simulink model "RL_sus_quarter_sim"  (R2025a)
settings: Solver=FixedStepAuto  StartTime=0.0  StopTime=20  FixedStep=0.001  RelTol=1e-3
model workspace (MAT data in the model file):
  G0 : Simulink.Parameter (value not decoded)
  Q_F : Simulink.Parameter (value not decoded)
  Q_dot_s : Simulink.Parameter (value not decoded)
  Q_dot_s_h : Simulink.Parameter (value not decoded)
  Q_dot_u : Simulink.Parameter (value not decoded)
  Q_flec : Simulink.Parameter (value not decoded)
  Q_flec_t : Simulink.Parameter (value not decoded)
  b_deflec : Simulink.Parameter (value not decoded)
  bump_height : Simulink.Parameter (value not decoded)
  bump_lenth : Simulink.Parameter (value not decoded)
  bump_start : Simulink.Parameter (value not decoded)
  f0 : Simulink.Parameter (value not decoded)
  kt : Simulink.Parameter (value not decoded)
  ms : Simulink.Parameter (value not decoded)
  n0 : Simulink.Parameter (value not decoded)
  n1 : Simulink.Parameter (value not decoded)
  omega_1 : Simulink.Parameter (value not decoded)
  omega_2 : Simulink.Parameter (value not decoded)
  omega_3 : Simulink.Parameter (value not decoded)
  omega_4 : Simulink.Parameter (value not decoded)
  ramp_height : Simulink.Parameter (value not decoded)
  ramp_lenth : Simulink.Parameter (value not decoded)
  ramp_start : Simulink.Parameter (value not decoded)
  sine_amp : Simulink.Parameter (value not decoded)
  sine_freq : Simulink.Parameter (value not decoded)
  u : Simulink.Parameter (value not decoded)
symbols that are objects in the model workspace (value not decoded): b_deflec, bump_height, bump_lenth, bump_start, f0, G0, kt, ms, n0, n1, omega_1, omega_2, omega_3, omega_4, Q_dot_s, Q_dot_s_h, Q_F, Q_flec, Q_flec_t, ramp_height, ramp_lenth, ramp_start, sine_amp, sine_freq
undefined symbols (not defined in the file): Ground, Hook, SH_ADD_new_as_as_xdef
libraries: fl_lib x250, nesl_utility x48, sharedTrackingLibrary x34, dspstat3 x18, simulink x3, deeplib x2, slpidlib x1
(part 7 of 12)

== system RL_sus_quarter_sim/Quarter_sys/Control/Y_1/freq semi/Subsystem2 ==
  v_def : Inport
  x_def : Inport  Port=2
  Add1 : Sum
  Gain : Gain  Gain=-1
  Lmbada_C : Constant  Value=1000
  Product1 : Product
  ks : Gain  Gain=-20000
  Out1 : Outport
  wires:
  ks/1 -> Add1/2
  x_def/1 -> ks/1
  Product1/1 -> Gain/1
  Lmbada_C/1 -> Product1/2
  Gain/1 -> Add1/1
  v_def/1 -> Product1/1
  Add1/1 -> Out1/1

== system RL_sus_quarter_sim/Quarter_sys/Control/Y_1/freq semi/Subsystem3 ==
  v_def : Inport
  x_def : Inport  Port=2
  Add1 : Sum
  Gain : Gain  Gain=-1
  Lmbada_C : Constant  Value=2000
  Product1 : Product
  ks : Gain  Gain=-20000
  Out1 : Outport
  wires:
  Add1/1 -> Out1/1
  v_def/1 -> Product1/1
  Gain/1 -> Add1/1
  Lmbada_C/1 -> Product1/2
  Product1/1 -> Gain/1
  x_def/1 -> ks/1
  ks/1 -> Add1/2

== system RL_sus_quarter_sim/Quarter_sys/Control/Y_1/imp_force_RL_model/Subsystem ==
  v_s : Inport
  Abs : Abs  SaturateOnIntegerOverflow=off
  Chart : Stateflow chart  TreatAsAtomicUnit=on  SystemSampleTime=0.001
  Chart1 : Stateflow chart  TreatAsAtomicUnit=on  SystemSampleTime=0.001
  Constant : Constant  Value=10000
  Constant1 : Constant  Value=10
  Constant2 : Constant  Value=1000
  Constant3 : Constant  Value=-500
  Constant4 : Constant  Value=-10000
  Constant5 : Constant  Value=30
  Constant6 : Constant  Value=3
  Constant8 : Constant  Value=0
  Demux : Demux  Outputs=2
  FS1 : Constant  Value=0.65
  FS2 : Constant  Value=4.5
  L1 : Subsystem
  L2 : Subsystem
  L3 : Subsystem
  MATLAB Function2 : Subsystem  Variant=on  VariantControlMode=label  VariantControl=MATLAB Function1  LabelModeActiveChoice=adaptive IFEKF simple
  Manual Switch : ManualSwitch
  Multiport Switch : MultiPortSwitch  Inputs=2  SaturateOnIntegerOverflow=off  InputSameDT=off
  Multiport Switch1 : MultiPortSwitch  Inputs=7  SaturateOnIntegerOverflow=off  InputSameDT=off
  Mux : Mux
  Mux1 : Mux  Inputs=2
  Mux2 : Mux  Inputs=2
  Scope : Scope
      settings: ActiveDisplayYMinimum=7.5  ActiveDisplayYMaximum=32.5
  Scope1 : Scope
      settings: ActiveDisplayYMinimum=-10696.7424  ActiveDisplayYMaximum=10249.86115  DataLoggingVariableName=ScopeData2
  Scope2 : Scope
      settings: ActiveDisplayYMinimum=0.875  ActiveDisplayYMaximum=2.125  DataLoggingVariableName=ScopeData3
  Zero-Order Hold : ZeroOrderHold  SampleTime=0.001
  passive : Subsystem
  Out1 : Outport
  wires:
  Constant8/1 -> MATLAB Function2/2(epsilon)
  Zero-Order Hold/1 -> MATLAB Function2/1(y)
  MATLAB Function2/6(omega) -> Abs/1
  v_s/1 -> Zero-Order Hold/1
  Abs/1 -> Chart/1(freq), Chart1/1(freq)
  FS1/1 -> Chart/2(FS1)
  FS2/1 -> Chart/3(FS2)
  Demux/1 -> Mux/1, Scope1/1  "k_a1"
  Constant3/1 -> Mux/2  "c_a1"
  Constant2/1 -> Mux/3  "c_a2"
  Demux/2 -> Scope/1, Mux/4  "b"
  Mux/1 -> ?
  Chart/1(level) -> Multiport Switch/1
  Multiport Switch/1 -> Demux/1
  Constant/1 -> Mux1/1  "ka1"
  Constant1/1 -> Mux1/2  "b"
  Mux1/1 -> Multiport Switch/2  "L1"
  Constant4/1 -> Mux2/1  "ka1"
  Constant5/1 -> Mux2/2  "b"
  Mux2/1 -> Multiport Switch/3  "L2"
  Chart1/1(level) -> Scope2/1, Manual Switch/1
  Multiport Switch1/1 -> Out1/1
  L1/1(Out1) -> Multiport Switch1/5, Multiport Switch1/8
  Manual Switch/1 -> Multiport Switch1/1
  Constant6/1 -> Manual Switch/2
  L3/1(Out1) -> Multiport Switch1/4, Multiport Switch1/7
  L2/1(Out1) -> Multiport Switch1/2, Multiport Switch1/3
  passive/1(Out1) -> Multiport Switch1/6

== system RL_sus_quarter_sim/Quarter_sys/Control/Y_1/imp_force_RL_model/bkkcc ==
  v_def : Inport
  x_def : Inport  Port=2
  a_def : Inport  Port=3
  param_ctr : Inport  Port=4
  Add : Sum  Inputs=+++
  Add1 : Sum
  Demux : Demux
  Divide : Product  Inputs=*/
  Gain{,1..3} (4 alike) : Gain  Gain=-1
  Integrator : Integrator
  Product{,1..3} (4 alike) : Product
  F_bkkcc : Outport
  wires:
  x_def/1 -> Product/2
  Demux/1 -> Gain/1  "k_a1"
  Product/1 -> Add/1
  Demux/2 -> Gain1/1  "c_a1"
  Product1/1 -> Add/2
  Add/1 -> F_bkkcc/1
  Demux/3 -> Product3/1, Gain2/1  "c_a2"
  Demux/4 -> Gain3/1  "b"
  Product2/1 -> Add/3
  Gain/1 -> Product/1
  Gain1/1 -> Product1/1
  Gain2/1 -> Product2/1
  Gain3/1 -> Divide/2
  param_ctr/1 -> Demux/1
  Add1/1 -> Integrator/1  "a1"
  Divide/1 -> Add1/1
  a_def/1 -> Add1/2
  v_def/1 -> Product1/2
  Integrator/1 -> Product2/2, Product3/2  "v1"
  Product3/1 -> Divide/1

== system RL_sus_quarter_sim/Quarter_sys/Passive/Y_1/P_0/Subsystem ==
  p0_k2 : Subsystem  VariantControl=p0_k2
  p0_k3 : Subsystem  VariantControl=p0_k3
  p0_k4 : Subsystem  VariantControl=p0_k4
  p0_k6 : Subsystem  VariantControl=p0_k6
  passive : Subsystem  VariantControl=passive
  Conn1 : PMIOPort  Side=Right
  Conn2 : PMIOPort  Port=2  Side=Left

== system RL_sus_quarter_sim/Quarter_sys/Passive/Y_1/P_1/Subsystem ==
  p1_k1 : Subsystem  VariantControl=p1_k1
  p1_k2 : Subsystem  VariantControl=p1_k2
  p1_k3 : Subsystem  VariantControl=p1_k3
  p1_k5 : Subsystem  VariantControl=p1_k5
  passive : Subsystem  VariantControl=passive
  Conn1 : PMIOPort  Side=Right
  Conn2 : PMIOPort  Port=2  Side=Left

== system RL_sus_quarter_sim/Quarter_sys/Passive/Y_1/P_test/Subsystem ==
  p1_k1 : Subsystem  VariantControl=p1_k1
  p1_k2 : Subsystem  VariantControl=p1_k2
  p1_k3 : Subsystem  VariantControl=p1_k3
  p1_k5 : Subsystem  VariantControl=p1_k5
  passive : Subsystem  VariantControl=passive
  Conn1 : PMIOPort  Side=Right
  Conn2 : PMIOPort  Port=2  Side=Left

== system RL_sus_quarter_sim/Quarter_sys/Passive/Y_1/Sky-Hook/Subsystem ==
  p1_k1 : Subsystem  VariantControl=p1_k1
  p1_k2 : Subsystem  VariantControl=p1_k2
  p1_k3 : Subsystem  VariantControl=p1_k3
  p1_k5 : Subsystem  VariantControl=p1_k5
  passive : Subsystem  VariantControl=passive
  Conn1 : PMIOPort  Side=Right
  Conn2 : PMIOPort  Port=2  Side=Left

== system RL_sus_quarter_sim/Quarter_sys/Control/Y_1/ADP_NN/reference/constant ==
  Add : Sum
  Constant : Constant  Value=0
  Constant1 : Constant  Value=0
  Constant2 : Constant  Value=sine_amp
  Manual Switch : ManualSwitch  CurrentSetting=0
  Repeating Sequence Stair : simulink/Sources/Repeating Sequence Stair  OutValues=[0 0.02].'  tsamp=3  OutMin=[]  OutMax=[]  OutDataTypeStr=double  OutputDataTypeScalingMode=double  OutDataType=fixdt(0,8)  ConRadixGroup=Best Precision: Vector-wise  OutScaling=2^-12
  xs_ref : Outport
  vs_ref : Outport  Port=2
  wires:
  Constant1/1 -> vs_ref/1
  Constant/1 -> Manual Switch/1
  Manual Switch/1 -> xs_ref/1
  Constant2/1 -> Add/1
  Repeating Sequence Stair/1 -> Add/2
  Add/1 -> Manual Switch/2

== system RL_sus_quarter_sim/Quarter_sys/Control/Y_1/ADP_NN/reference/skyhook_virtual ==
  xs : Inport
  vs : Inport  Port=2
  Add : Sum
  Add1 : Sum
  Add2 : Sum
  Divide : Product  Inputs=*/
  Product : Product
  Product1 : Product
  dt_v : Gain  Gain=0.1
  ms_v : Constant  Value=400
  skyhook_c : Constant  Value=-1000
  skyhook_k : Constant  Value=-10000
  xs_ref : Outport
  vs_ref : Outport  Port=2
  wires:
  xs/1 -> Add1/2, Product/1
  skyhook_k/1 -> Product/2
  vs/1 -> Add2/2, Product1/1
  skyhook_c/1 -> Product1/2
  Product/1 -> Add/1
  Product1/1 -> Add/2
  Add/1 -> Divide/1  "F_skyhook_v"
  ms_v/1 -> Divide/2
  Divide/1 -> dt_v/1  "skyhook_as_v"
  dt_v/1 -> Add2/1, Add1/1
  Add1/1 -> xs_ref/1
  Add2/1 -> vs_ref/1

== system RL_sus_quarter_sim/Quarter_sys/Control/Y_1/Freq_imp/Low_with_Alpha/Subsystem ==
  p1_k1 : Subsystem  VariantControl=p1_k1
  p1_k2 : Subsystem  VariantControl=p1_k2
  p1_k3 : Subsystem  VariantControl=p1_k3
  p1_k5 : Subsystem  VariantControl=p1_k5
  passive : Subsystem  VariantControl=passive
  Conn1 : PMIOPort  Side=Right
  Conn2 : PMIOPort  Port=2  Side=Left

== system RL_sus_quarter_sim/Quarter_sys/Control/Y_1/Freq_imp/high_with_Alpha/Subsystem ==
  p1_k1 : Subsystem  VariantControl=p1_k1
  p1_k2 : Subsystem  VariantControl=p1_k2
  p1_k3 : Subsystem  VariantControl=p1_k3
  p1_k5 : Subsystem  VariantControl=p1_k5
  passive : Subsystem  VariantControl=passive
  Conn1 : PMIOPort  Side=Right
  Conn2 : PMIOPort  Port=2  Side=Left

== system RL_sus_quarter_sim/Quarter_sys/Control/Y_1/Freq_imp1/Low_with_Alpha/Subsystem ==
  p1_k1 : Subsystem  VariantControl=p1_k1
  p1_k2 : Subsystem  VariantControl=p1_k2
  p1_k3 : Subsystem  VariantControl=p1_k3
  p1_k5 : Subsystem  VariantControl=p1_k5
  passive : Subsystem  VariantControl=passive
  Conn1 : PMIOPort  Side=Right
  Conn2 : PMIOPort  Port=2  Side=Left

== system RL_sus_quarter_sim/Quarter_sys/Control/Y_1/Freq_imp1/Subsystem/2nd_FS ==
  vs : Inport
  au : Inport  Port=2
  alpha : Inport  Port=3
  2nd_FS : Sum  Inputs=+-
  Constant4 : Constant  Value=20000
  Constant5 : Constant  Value=400
  Constant6 : Constant  Value=1000
  Gain : Gain  Gain=2*pi
  MATLAB Function1 : MATLAB Function  TreatAsAtomicUnit=on
  Product : Product
  Square : Math  Operator=square
  Square1 : Math  Operator=square
  FS2 : Outport
  wires:
  Gain/1 -> Square/1, MATLAB Function1/2(alpha)
  Square/1 -> Product/1
  Constant5/1 -> MATLAB Function1/4(ms)
  2nd_FS/1 -> FS2/1
  MATLAB Function1/1(y) -> 2nd_FS/1
  Constant6/1 -> MATLAB Function1/5(cs)
  Constant4/1 -> MATLAB Function1/3(ks)
  Product/1 -> 2nd_FS/2
  au/1 -> MATLAB Function1/1(au)
  vs/1 -> Square1/1
  Square1/1 -> Product/2
  alpha/1 -> Gain/1

== system RL_sus_quarter_sim/Quarter_sys/Control/Y_1/Freq_imp1/Subsystem/FS1 ==
  vs : Inport
  au : Inport  Port=2
  alpha : Inport  Port=3
  2nd_FS : Sum  Inputs=+-
  Constant4 : Constant  Value=20000
  Constant5 : Constant  Value=400
  Constant6 : Constant  Value=1000
  Gain : Gain  Gain=2*pi
  MATLAB Function1 : MATLAB Function  TreatAsAtomicUnit=on
  Product : Product
  Scope : Scope  NumInputPorts=2
      settings: ActiveDisplayYMinimum=-2.36691  ActiveDisplayYMaximum=3.61329  DataLoggingVariableName=ScopeData8
  Square : Math  Operator=square
  Square1 : Math  Operator=square
  FS2 : Outport
  wires:
  Square1/1 -> Product/2
  vs/1 -> Square1/1
  au/1 -> MATLAB Function1/1(au)
  Product/1 -> Scope/2, 2nd_FS/2
  Constant4/1 -> MATLAB Function1/3(ks)
  Constant6/1 -> MATLAB Function1/5(cs)
  MATLAB Function1/1(y) -> Scope/1, 2nd_FS/1
  2nd_FS/1 -> FS2/1
  Constant5/1 -> MATLAB Function1/4(ms)
  Square/1 -> Product/1
  Gain/1 -> MATLAB Function1/2(alpha), Square/1
  alpha/1 -> Gain/1

== system RL_sus_quarter_sim/Quarter_sys/Control/Y_1/Freq_imp1/high_with_Alpha/Subsystem ==
  p1_k1 : Subsystem  VariantControl=p1_k1
  p1_k2 : Subsystem  VariantControl=p1_k2
  p1_k3 : Subsystem  VariantControl=p1_k3
  p1_k5 : Subsystem  VariantControl=p1_k5
  passive : Subsystem  VariantControl=passive
  Conn1 : PMIOPort  Side=Right
  Conn2 : PMIOPort  Port=2  Side=Left

== system RL_sus_quarter_sim/Quarter_sys/Control/Y_1/IFEKF FDC/Subsystem/MATLAB Function2 ==
  y : Inport
  epsilon : Inport  Port=2
  EKF epsilon : Subsystem  VariantControl=Extended Kalman Filter habib epsilon
  EKF simple Amp : Subsystem  VariantControl=EKFhabib epsilon Amp
  IFEKF simple : Subsystem  VariantControl=IFEKF simple
  adaptive IFEKF sdimple_3 : Subsystem  VariantControl=adaptive IFEKF sdimple_3
  adaptive IFEKF simple : Subsystem  VariantControl=adaptive IFEKF simple
  x1hat : Outport
  P : Outport  Port=2
  debug : Outport  Port=3
  xhat_pred : Outport  Port=4
  y_residual : Outport  Port=5
  omega : Outport  Port=6

== system RL_sus_quarter_sim/Quarter_sys/Control/Y_1/IFEKF SHADD/Subsystem/MATLAB Function2 ==
  y : Inport
  epsilon : Inport  Port=2
  EKF epsilon : Subsystem  VariantControl=Extended Kalman Filter habib epsilon
  EKF simple Amp : Subsystem  VariantControl=EKFhabib epsilon Amp
  IFEKF simple : Subsystem  VariantControl=IFEKF simple
  adaptive IFEKF simple : Subsystem  VariantControl=adaptive IFEKF simple
  x1hat : Outport
  P : Outport  Port=2
  debug : Outport  Port=3
  xhat_pred : Outport  Port=4
  y_residual : Outport  Port=5
  omega : Outport  Port=6

== system RL_sus_quarter_sim/Quarter_sys/Control/Y_1/IFEKF Select c/Subsystem/MATLAB Function2 ==
  y : Inport
  epsilon : Inport  Port=2
  EKF epsilon : Subsystem  VariantControl=Extended Kalman Filter habib epsilon
  EKF simple Amp : Subsystem  VariantControl=EKFhabib epsilon Amp
  IFEKF simple : Subsystem  VariantControl=IFEKF simple
  adaptive IFEKF simple : Subsystem  VariantControl=adaptive IFEKF simple
  x1hat : Outport
  P : Outport  Port=2
  debug : Outport  Port=3
  xhat_pred : Outport  Port=4
  y_residual : Outport  Port=5
  omega : Outport  Port=6

== system RL_sus_quarter_sim/Quarter_sys/Control/Y_1/IFEKF Select c/Subsystem2/constant ==
  sig select : Inport
  v_def : Inport  Port=2
  Multiport Switch : MultiPortSwitch  SaturateOnIntegerOverflow=off  InputSameDT=off
  large C : Subsystem
  "mid C " : Subsystem
  small C : Subsystem
  F_damper : Outport
  wires:
  Multiport Switch/1 -> F_damper/1  "F_damper"
  small C/1(Out1) -> Multiport Switch/3
  large C/1(F_sus1) -> Multiport Switch/2
  "mid C "/1(Out1) -> Multiport Switch/4
  sig select/1 -> Multiport Switch/1
  v_def/1 -> large C/1(v_def), "mid C "/1(v_def), small C/1(v_def)

== system RL_sus_quarter_sim/Quarter_sys/Control/Y_1/IFEKF Select c/Subsystem2/semi ctr ==
  sig select : Inport
  v_def : Inport  Port=2
  v_s : Inport  Port=3
  a_s : Inport  Port=4
  ADD : Subsystem
  Multiport Switch : MultiPortSwitch  SaturateOnIntegerOverflow=off  InputSameDT=off
  SH : Subsystem
  Subsystem1 : Subsystem
  F_damper : Outport
  wires:
  v_s/1 -> SH/2(v_s)
  v_def/1 -> SH/1(v_def), Subsystem1/1(v_def), ADD/1(v_def)
  sig select/1 -> Multiport Switch/1
  Subsystem1/1(Out1) -> Multiport Switch/4
  ADD/1(F_sus1) -> Multiport Switch/3
  a_s/1 -> ADD/2(a_s)
  SH/1(Out1) -> Multiport Switch/2
  Multiport Switch/1 -> F_damper/1  "F_damper"

== system RL_sus_quarter_sim/Quarter_sys/Control/Y_1/IFEKF freq b/Subsystem/MATLAB Function2 ==
  y : Inport
  epsilon : Inport  Port=2
  EKF epsilon : Subsystem  VariantControl=Extended Kalman Filter habib epsilon
  EKF simple Amp : Subsystem  VariantControl=EKFhabib epsilon Amp
  IFEKF simple : Subsystem  VariantControl=IFEKF simple
  adaptive IFEKF simple : Subsystem  VariantControl=adaptive IFEKF simple
  x1hat : Outport
  P : Outport  Port=2
  debug : Outport  Port=3
  xhat_pred : Outport  Port=4
  y_residual : Outport  Port=5
  omega : Outport  Port=6

== system RL_sus_quarter_sim/Quarter_sys/Control/Y_1/IFEKF freq bc/Subsystem/MATLAB Function2 ==
  y : Inport
  epsilon : Inport  Port=2
  EKF epsilon : Subsystem  VariantControl=Extended Kalman Filter habib epsilon
  EKF simple Amp : Subsystem  VariantControl=EKFhabib epsilon Amp
  IFEKF simple : Subsystem  VariantControl=IFEKF simple
  adaptive IFEKF simple : Subsystem  VariantControl=adaptive IFEKF simple
  x1hat : Outport
  P : Outport  Port=2
  debug : Outport  Port=3
  xhat_pred : Outport  Port=4
  y_residual : Outport  Port=5
  omega : Outport  Port=6

== system RL_sus_quarter_sim/Quarter_sys/Control/Y_1/IFEKF freq bkkcc/Subsystem/L1 ==
  Constant1 : Constant  Value=0.5
  Constant2 : Constant  Value=1000
  Constant3 : Constant  Value=-500
  Constant4 : Constant  Value=10000
  Mux : Mux
  Out1 : Outport
  wires:
  Mux/1 -> Out1/1
  Constant3/1 -> Mux/2  "c_a1"
  Constant2/1 -> Mux/3  "c_a2"
  Constant4/1 -> Mux/1  "k_a1"
  Constant1/1 -> Mux/4  "b"

== system RL_sus_quarter_sim/Quarter_sys/Control/Y_1/IFEKF freq bkkcc/Subsystem/L2 ==
  Constant1 : Constant  Value=30
  Constant2 : Constant  Value=1000
  Constant3 : Constant  Value=-500
  Constant4 : Constant  Value=-10000
  Mux : Mux
  Out1 : Outport
  wires:
  Constant1/1 -> Mux/4  "b"
  Constant4/1 -> Mux/1  "k_a1"
  Constant2/1 -> Mux/3  "c_a2"
  Constant3/1 -> Mux/2  "c_a1"
  Mux/1 -> Out1/1

== system RL_sus_quarter_sim/Quarter_sys/Control/Y_1/IFEKF freq bkkcc/Subsystem/L3 ==
  Constant1 : Constant  Value=10
  Constant2 : Constant  Value=1000
  Constant3 : Constant  Value=-500
  Constant4 : Constant  Value=-10000
  Mux : Mux
  Out1 : Outport
  wires:
  Constant1/1 -> Mux/4  "b"
  Constant4/1 -> Mux/1  "k_a1"
  Constant2/1 -> Mux/3  "c_a2"
  Constant3/1 -> Mux/2  "c_a1"
  Mux/1 -> Out1/1

== system RL_sus_quarter_sim/Quarter_sys/Control/Y_1/IFEKF freq bkkcc/Subsystem/MATLAB Function2 ==
  y : Inport
  epsilon : Inport  Port=2
  EKF epsilon : Subsystem  VariantControl=Extended Kalman Filter habib epsilon
  EKF simple Amp : Subsystem  VariantControl=EKFhabib epsilon Amp
  IFEKF simple : Subsystem  VariantControl=IFEKF simple
  adaptive IFEKF simple : Subsystem  VariantControl=adaptive IFEKF simple
  x1hat : Outport
  P : Outport  Port=2
  debug : Outport  Port=3
  xhat_pred : Outport  Port=4
  y_residual : Outport  Port=5
  omega : Outport  Port=6

== system RL_sus_quarter_sim/Quarter_sys/Control/Y_1/IFEKF freq bkkcc/Subsystem/passive ==
  Constant1 : Constant  Value=20
  Constant2 : Constant  Value=0
  Constant3 : Constant  Value=0
  Constant4 : Constant  Value=0
  Mux : Mux
  Out1 : Outport
  wires:
  Mux/1 -> Out1/1
  Constant3/1 -> Mux/2  "c_a1"
  Constant2/1 -> Mux/3  "c_a2"
  Constant4/1 -> Mux/1  "k_a1"
  Constant1/1 -> Mux/4  "b"

== system RL_sus_quarter_sim/Quarter_sys/Control/Y_1/IFEKF freq bkkcc/Subsystem1/Subsystem1 ==
  b : fl_lib/Mechanical/Translational Elements/Translational Inerter  B=10 kg  v_specify=off  v_priority=High  v=0 m/s  v_nominal_specify=off  v_nominal_value=1  v_nominal_unit=m/s  f_specify=off  f_priority=None  f=0 N  f_nominal_specify=off  f_nominal_value=1  f_nominal_unit=N
      settings: InternalSimscapePortConfiguration="{\"Bottom\":[],\"Left\":[{\"id\":\"R\",\"label\":\"R\",\"type\":\"foundation.mechanical.translational.translational\"}],\"Right\":[{\"id\":\"C\",\"label\":\"C\",\"type\":\"foundation.mechanical.translational.translational\"}],\"Top\":[]}"
  c_a2 : fl_lib/Mechanical/Translational Elements/Translational Damper  D=1000 N*s/m  v_specify=off  v_priority=None  v=0 m/s  v_nominal_specify=off  v_nominal_value=1  v_nominal_unit=m/s  f_specify=off  f_priority=None  f=0 N  f_nominal_specify=off  f_nominal_value=1  f_nominal_unit=N
  Conn1 : PMIOPort  Side=Right
  Conn2 : PMIOPort  Port=2  Side=Left
  connections:
  Conn1/RConn1 -- c_a2/RConn1
  b/LConn1 -- Conn2/RConn1
  c_a2/LConn1 -- b/RConn1

== system RL_sus_quarter_sim/Quarter_sys/Control/Y_1/IFEKF freq c/Subsystem/MATLAB Function2 ==
  y : Inport
  epsilon : Inport  Port=2
  EKF epsilon : Subsystem  VariantControl=Extended Kalman Filter habib epsilon
  EKF simple Amp : Subsystem  VariantControl=EKFhabib epsilon Amp
  IFEKF simple : Subsystem  VariantControl=IFEKF simple
  adaptive IFEKF simple : Subsystem  VariantControl=adaptive IFEKF simple
  x1hat : Outport
  P : Outport  Port=2
  debug : Outport  Port=3
  xhat_pred : Outport  Port=4
  y_residual : Outport  Port=5
  omega : Outport  Port=6

== system RL_sus_quarter_sim/Quarter_sys/Control/Y_1/PA bk/Subsystem/Subsystem1 ==
  Translational Inerter : fl_lib/Mechanical/Translational Elements/Translational Inerter  B=10 kg  v_specify=off  v_priority=High  v=0 m/s  v_nominal_specify=off  v_nominal_value=1  v_nominal_unit=m/s  f_specify=off  f_priority=None  f=0 N  f_nominal_specify=off  f_nominal_value=1  f_nominal_unit=N
      settings: InternalSimscapePortConfiguration="{\"Bottom\":[],\"Left\":[{\"id\":\"R\",\"label\":\"R\",\"type\":\"foundation.mechanical.translational.translational\"}],\"Right\":[{\"id\":\"C\",\"label\":\"C\",\"type\":\"foundation.mechanical.translational.translational\"}],\"Top\":[]}"
  Translational Spring1 : fl_lib/Mechanical/Translational Elements/Translational Spring  spr_rate=2000 N/m  v_specify=off  v_priority=None  v=0 m/s  v_nominal_specify=off  v_nominal_value=1  v_nominal_unit=m/s  f_specify=off  f_priority=None  f=0 N  f_nominal_specify=off  f_nominal_value=1  f_nominal_unit=N  x_specify=off  x_priority=High  x=0 m  x_nominal_specify=off  x_nominal_value=1  x_nominal_unit=m
  Conn1 : PMIOPort  Side=Right
  Conn2 : PMIOPort  Port=2  Side=Left
  connections:
  Conn1/RConn1 -- Translational Spring1/RConn1
  Translational Inerter/LConn1 -- Conn2/RConn1
  Translational Spring1/LConn1 -- Translational Inerter/RConn1

== system RL_sus_quarter_sim/Quarter_sys/Control/Y_1/PA bkc/Subsystem/Subsystem1 ==
  Translational Inerter : fl_lib/Mechanical/Translational Elements/Translational Inerter  B=10 kg  v_specify=off  v_priority=High  v=0 m/s  v_nominal_specify=off  v_nominal_value=1  v_nominal_unit=m/s  f_specify=off  f_priority=None  f=0 N  f_nominal_specify=off  f_nominal_value=1  f_nominal_unit=N
      settings: InternalSimscapePortConfiguration="{\"Bottom\":[],\"Left\":[{\"id\":\"R\",\"label\":\"R\",\"type\":\"foundation.mechanical.translational.translational\"}],\"Right\":[{\"id\":\"C\",\"label\":\"C\",\"type\":\"foundation.mechanical.translational.translational\"}],\"Top\":[]}"
  Translational Damper : fl_lib/Mechanical/Translational Elements/Translational Damper  D=100 N*s/m  v_specify=off  v_priority=None  v=0 m/s  v_nominal_specify=off  v_nominal_value=1  v_nominal_unit=m/s  f_specify=off  f_priority=None  f=0 N  f_nominal_specify=off  f_nominal_value=1  f_nominal_unit=N
  Translational Spring1 : fl_lib/Mechanical/Translational Elements/Translational Spring  spr_rate=5000 N/m  v_specify=off  v_priority=None  v=0 m/s  v_nominal_specify=off  v_nominal_value=1  v_nominal_unit=m/s  f_specify=off  f_priority=None  f=0 N  f_nominal_specify=off  f_nominal_value=1  f_nominal_unit=N  x_specify=off  x_priority=High  x=0 m  x_nominal_specify=off  x_nominal_value=1  x_nominal_unit=m
  Conn1 : PMIOPort  Side=Right
  Conn2 : PMIOPort  Port=2  Side=Left
  connections:
  Translational Spring1/LConn1 -- Translational Damper/LConn1 -- Translational Inerter/RConn1
  Translational Inerter/LConn1 -- Conn2/RConn1
  Conn1/RConn1 -- Translational Spring1/RConn1 -- Translational Damper/RConn1

== system RL_sus_quarter_sim/Quarter_sys/Control/Y_1/PA bkkcc/Subsystem/Subsystem1 ==
  b : fl_lib/Mechanical/Translational Elements/Translational Inerter  B=10 kg  v_specify=off  v_priority=High  v=0 m/s  v_nominal_specify=off  v_nominal_value=1  v_nominal_unit=m/s  f_specify=off  f_priority=None  f=0 N  f_nominal_specify=off  f_nominal_value=1  f_nominal_unit=N
      settings: InternalSimscapePortConfiguration="{\"Bottom\":[],\"Left\":[{\"id\":\"R\",\"label\":\"R\",\"type\":\"foundation.mechanical.translational.translational\"}],\"Right\":[{\"id\":\"C\",\"label\":\"C\",\"type\":\"foundation.mechanical.translational.translational\"}],\"Top\":[]}"
  c_a2 : fl_lib/Mechanical/Translational Elements/Translational Damper  D=1000 N*s/m  v_specify=off  v_priority=None  v=0 m/s  v_nominal_specify=off  v_nominal_value=1  v_nominal_unit=m/s  f_specify=off  f_priority=None  f=0 N  f_nominal_specify=off  f_nominal_value=1  f_nominal_unit=N
  Conn1 : PMIOPort  Side=Right
  Conn2 : PMIOPort  Port=2  Side=Left
  connections:
  Conn1/RConn1 -- c_a2/RConn1
  b/LConn1 -- Conn2/RConn1
  c_a2/LConn1 -- b/RConn1

== system RL_sus_quarter_sim/Quarter_sys/Control/Y_1/P_0/Subsystem/p0_k2 ==
  Translational Inerter : fl_lib/Mechanical/Translational Elements/Translational Inerter  B=1 kg  v_specify=off  v_priority=High  v=0 m/s  v_nominal_specify=off  v_nominal_value=1  v_nominal_unit=m/s  f_specify=off  f_priority=None  f=0 N  f_nominal_specify=off  f_nominal_value=1  f_nominal_unit=N
      settings: InternalSimscapePortConfiguration="{\"Bottom\":[],\"Left\":[{\"id\":\"R\",\"label\":\"R\",\"type\":\"foundation.mechanical.translational.translational\"}],\"Right\":[{\"id\":\"C\",\"label\":\"C\",\"type\":\"foundation.mechanical.translational.translational\"}],\"Top\":[]}"
  Translational Damper : fl_lib/Mechanical/Translational Elements/Translational Damper  D=2000 N*s/m  v_specify=off  v_priority=None  v=0 m/s  v_nominal_specify=off  v_nominal_value=1  v_nominal_unit=m/s  f_specify=off  f_priority=None  f=0 N  f_nominal_specify=off  f_nominal_value=1  f_nominal_unit=N
  Translational Spring1 : fl_lib/Mechanical/Translational Elements/Translational Spring  spr_rate=20000 N/m  v_specify=off  v_priority=None  v=0 m/s  v_nominal_specify=off  v_nominal_value=1  v_nominal_unit=m/s  f_specify=off  f_priority=None  f=0 N  f_nominal_specify=off  f_nominal_value=1  f_nominal_unit=N  x_specify=off  x_priority=High  x=0 m  x_nominal_specify=off  x_nominal_value=1  x_nominal_unit=m
  Conn1 : PMIOPort  Side=Right
  Conn2 : PMIOPort  Port=2  Side=Left
  connections:
  Translational Spring1/LConn1 -- Translational Damper/RConn1 -- Translational Inerter/LConn1
  Conn1/RConn1 -- Translational Inerter/RConn1 -- Translational Spring1/RConn1
  Translational Damper/LConn1 -- Conn2/RConn1

== system RL_sus_quarter_sim/Quarter_sys/Control/Y_1/P_0/Subsystem/p0_k3 ==
  Translational Inerter : fl_lib/Mechanical/Translational Elements/Translational Inerter  B=1 kg  v_specify=off  v_priority=High  v=0 m/s  v_nominal_specify=off  v_nominal_value=1  v_nominal_unit=m/s  f_specify=off  f_priority=None  f=0 N  f_nominal_specify=off  f_nominal_value=1  f_nominal_unit=N
      settings: InternalSimscapePortConfiguration="{\"Bottom\":[],\"Left\":[{\"id\":\"R\",\"label\":\"R\",\"type\":\"foundation.mechanical.translational.translational\"}],\"Right\":[{\"id\":\"C\",\"label\":\"C\",\"type\":\"foundation.mechanical.translational.translational\"}],\"Top\":[]}"
  Translational Damper : fl_lib/Mechanical/Translational Elements/Translational Damper  D=2000 N*s/m  v_specify=off  v_priority=None  v=0 m/s  v_nominal_specify=off  v_nominal_value=1  v_nominal_unit=m/s  f_specify=off  f_priority=None  f=0 N  f_nominal_specify=off  f_nominal_value=1  f_nominal_unit=N
  Translational Spring1 : fl_lib/Mechanical/Translational Elements/Translational Spring  spr_rate=20000 N/m  v_specify=off  v_priority=None  v=0 m/s  v_nominal_specify=off  v_nominal_value=1  v_nominal_unit=m/s  f_specify=off  f_priority=None  f=0 N  f_nominal_specify=off  f_nominal_value=1  f_nominal_unit=N  x_specify=off  x_priority=High  x=0 m  x_nominal_specify=off  x_nominal_value=1  x_nominal_unit=m
  Conn1 : PMIOPort  Side=Right
  Conn2 : PMIOPort  Port=2  Side=Left
  connections:
  Conn1/RConn1 -- Translational Spring1/RConn1
  Translational Spring1/LConn1 -- Translational Inerter/RConn1
  Conn2/RConn1 -- Translational Damper/LConn1
  Translational Damper/RConn1 -- Translational Inerter/LConn1

== system RL_sus_quarter_sim/Quarter_sys/Control/Y_1/P_0/Subsystem/p0_k4 ==
  Translational Inerter : fl_lib/Mechanical/Translational Elements/Translational Inerter  B=1 kg  v_specify=off  v_priority=High  v=0 m/s  v_nominal_specify=off  v_nominal_value=1  v_nominal_unit=m/s  f_specify=off  f_priority=None  f=0 N  f_nominal_specify=off  f_nominal_value=1  f_nominal_unit=N
      settings: InternalSimscapePortConfiguration="{\"Bottom\":[],\"Left\":[{\"id\":\"R\",\"label\":\"R\",\"type\":\"foundation.mechanical.translational.translational\"}],\"Right\":[{\"id\":\"C\",\"label\":\"C\",\"type\":\"foundation.mechanical.translational.translational\"}],\"Top\":[]}"
  Translational Damper : fl_lib/Mechanical/Translational Elements/Translational Damper  D=2000 N*s/m  v_specify=off  v_priority=None  v=0 m/s  v_nominal_specify=off  v_nominal_value=1  v_nominal_unit=m/s  f_specify=off  f_priority=None  f=0 N  f_nominal_specify=off  f_nominal_value=1  f_nominal_unit=N
  Translational Spring1 : fl_lib/Mechanical/Translational Elements/Translational Spring  spr_rate=20000 N/m  v_specify=off  v_priority=None  v=0 m/s  v_nominal_specify=off  v_nominal_value=1  v_nominal_unit=m/s  f_specify=off  f_priority=None  f=0 N  f_nominal_specify=off  f_nominal_value=1  f_nominal_unit=N  x_specify=off  x_priority=High  x=0 m  x_nominal_specify=off  x_nominal_value=1  x_nominal_unit=m
  Conn1 : PMIOPort  Side=Right
  Conn2 : PMIOPort  Port=2  Side=Left
  connections:
  Translational Spring1/RConn1 -- Translational Inerter/LConn1 -- Translational Damper/RConn1
  Translational Spring1/LConn1 -- Translational Damper/LConn1 -- Conn2/RConn1
  Translational Inerter/RConn1 -- Conn1/RConn1

== system RL_sus_quarter_sim/Quarter_sys/Control/Y_1/P_0/Subsystem/p0_k6 ==
  Translational Inerter : fl_lib/Mechanical/Translational Elements/Translational Inerter  B=1 kg  v_specify=off  v_priority=High  v=0 m/s  v_nominal_specify=off  v_nominal_value=1  v_nominal_unit=m/s  f_specify=off  f_priority=None  f=0 N  f_nominal_specify=off  f_nominal_value=1  f_nominal_unit=N
      settings: InternalSimscapePortConfiguration="{\"Bottom\":[],\"Left\":[{\"id\":\"R\",\"label\":\"R\",\"type\":\"foundation.mechanical.translational.translational\"}],\"Right\":[{\"id\":\"C\",\"label\":\"C\",\"type\":\"foundation.mechanical.translational.translational\"}],\"Top\":[]}"
  Translational Damper : fl_lib/Mechanical/Translational Elements/Translational Damper  D=2000 N*s/m  v_specify=off  v_priority=None  v=0 m/s  v_nominal_specify=off  v_nominal_value=1  v_nominal_unit=m/s  f_specify=off  f_priority=None  f=0 N  f_nominal_specify=off  f_nominal_value=1  f_nominal_unit=N
  Translational Spring1 : fl_lib/Mechanical/Translational Elements/Translational Spring  spr_rate=20000 N/m  v_specify=off  v_priority=None  v=0 m/s  v_nominal_specify=off  v_nominal_value=1  v_nominal_unit=m/s  f_specify=off  f_priority=None  f=0 N  f_nominal_specify=off  f_nominal_value=1  f_nominal_unit=N  x_specify=off  x_priority=High  x=0 m  x_nominal_specify=off  x_nominal_value=1  x_nominal_unit=m
  Conn1 : PMIOPort  Side=Right
  Conn2 : PMIOPort  Port=2  Side=Left
  connections:
  Translational Damper/RConn1 -- Translational Inerter/LConn1
  Conn1/RConn1 -- Translational Spring1/RConn1 -- Translational Inerter/RConn1
  Conn2/RConn1 -- Translational Damper/LConn1 -- Translational Spring1/LConn1

== system RL_sus_quarter_sim/Quarter_sys/Control/Y_1/P_0/Subsystem/passive ==
  Translational Damper : fl_lib/Mechanical/Translational Elements/Translational Damper  D=2000 N*s/m  v_specify=off  v_priority=None  v=0 m/s  v_nominal_specify=off  v_nominal_value=1  v_nominal_unit=m/s  f_specify=off  f_priority=None  f=0 N  f_nominal_specify=off  f_nominal_value=1  f_nominal_unit=N
  Translational Spring1 : fl_lib/Mechanical/Translational Elements/Translational Spring  spr_rate=200000 N/m  v_specify=off  v_priority=None  v=0 m/s  v_nominal_specify=off  v_nominal_value=1  v_nominal_unit=m/s  f_specify=off  f_priority=None  f=0 N  f_nominal_specify=off  f_nominal_value=1  f_nominal_unit=N  x_specify=off  x_priority=High  x=0 m  x_nominal_specify=off  x_nominal_value=1  x_nominal_unit=m
  Conn1 : PMIOPort  Side=Right
  Conn2 : PMIOPort  Port=2  Side=Left
  connections:
  Translational Damper/RConn1 -- Translational Spring1/RConn1 -- Conn1/RConn1
  Conn2/RConn1 -- Translational Damper/LConn1 -- Translational Spring1/LConn1

== system RL_sus_quarter_sim/Quarter_sys/Control/Y_1/P_1/Subsystem/p1_k1 ==
  Translational Inerter : fl_lib/Mechanical/Translational Elements/Translational Inerter  B=1 kg  v_specify=off  v_priority=High  v=0 m/s  v_nominal_specify=off  v_nominal_value=1  v_nominal_unit=m/s  f_specify=off  f_priority=None  f=0 N  f_nominal_specify=off  f_nominal_value=1  f_nominal_unit=N
      settings: InternalSimscapePortConfiguration="{\"Bottom\":[],\"Left\":[{\"id\":\"R\",\"label\":\"R\",\"type\":\"foundation.mechanical.translational.translational\"}],\"Right\":[{\"id\":\"C\",\"label\":\"C\",\"type\":\"foundation.mechanical.translational.translational\"}],\"Top\":[]}"
  Translational Damper : fl_lib/Mechanical/Translational Elements/Translational Damper  D=2000 N*s/m  v_specify=off  v_priority=None  v=0 m/s  v_nominal_specify=off  v_nominal_value=1  v_nominal_unit=m/s  f_specify=off  f_priority=None  f=0 N  f_nominal_specify=off  f_nominal_value=1  f_nominal_unit=N
  Translational Spring1 : fl_lib/Mechanical/Translational Elements/Translational Spring  spr_rate=20000 N/m  v_specify=off  v_priority=None  v=0 m/s  v_nominal_specify=off  v_nominal_value=1  v_nominal_unit=m/s  f_specify=off  f_priority=None  f=0 N  f_nominal_specify=off  f_nominal_value=1  f_nominal_unit=N  x_specify=off  x_priority=High  x=0 m  x_nominal_specify=off  x_nominal_value=1  x_nominal_unit=m
  Conn1 : PMIOPort  Side=Right
  Conn2 : PMIOPort  Port=2  Side=Left
  connections:
  Conn1/RConn1 -- Translational Damper/RConn1 -- Translational Spring1/RConn1
  Translational Spring1/LConn1 -- Translational Inerter/RConn1
  Conn2/RConn1 -- Translational Damper/LConn1 -- Translational Inerter/LConn1

== system RL_sus_quarter_sim/Quarter_sys/Control/Y_1/P_1/Subsystem/p1_k2 ==
  Translational Inerter : fl_lib/Mechanical/Translational Elements/Translational Inerter  B=1 kg  v_specify=off  v_priority=High  v=0 m/s  v_nominal_specify=off  v_nominal_value=1  v_nominal_unit=m/s  f_specify=off  f_priority=None  f=0 N  f_nominal_specify=off  f_nominal_value=1  f_nominal_unit=N
      settings: InternalSimscapePortConfiguration="{\"Bottom\":[],\"Left\":[{\"id\":\"R\",\"label\":\"R\",\"type\":\"foundation.mechanical.translational.translational\"}],\"Right\":[{\"id\":\"C\",\"label\":\"C\",\"type\":\"foundation.mechanical.translational.translational\"}],\"Top\":[]}"
  Translational Damper : fl_lib/Mechanical/Translational Elements/Translational Damper  D=2000 N*s/m  v_specify=off  v_priority=None  v=0 m/s  v_nominal_specify=off  v_nominal_value=1  v_nominal_unit=m/s  f_specify=off  f_priority=None  f=0 N  f_nominal_specify=off  f_nominal_value=1  f_nominal_unit=N
  Translational Spring1 : fl_lib/Mechanical/Translational Elements/Translational Spring  spr_rate=20000 N/m  v_specify=off  v_priority=None  v=0 m/s  v_nominal_specify=off  v_nominal_value=1  v_nominal_unit=m/s  f_specify=off  f_priority=None  f=0 N  f_nominal_specify=off  f_nominal_value=1  f_nominal_unit=N  x_specify=off  x_priority=High  x=0 m  x_nominal_specify=off  x_nominal_value=1  x_nominal_unit=m
  Conn1 : PMIOPort  Side=Right
  Conn2 : PMIOPort  Port=2  Side=Left
  connections:
  Translational Inerter/LConn1 -- Translational Damper/LConn1 -- Conn2/RConn1
  Translational Spring1/RConn1 -- Translational Inerter/RConn1 -- Conn1/RConn1
  Translational Spring1/LConn1 -- Translational Damper/RConn1

== system RL_sus_quarter_sim/Quarter_sys/Control/Y_1/P_1/Subsystem/p1_k3 ==
  Translational Inerter : fl_lib/Mechanical/Translational Elements/Translational Inerter  B=1 kg  v_specify=off  v_priority=High  v=0 m/s  v_nominal_specify=off  v_nominal_value=1  v_nominal_unit=m/s  f_specify=off  f_priority=None  f=0 N  f_nominal_specify=off  f_nominal_value=1  f_nominal_unit=N
      settings: InternalSimscapePortConfiguration="{\"Bottom\":[],\"Left\":[{\"id\":\"R\",\"label\":\"R\",\"type\":\"foundation.mechanical.translational.translational\"}],\"Right\":[{\"id\":\"C\",\"label\":\"C\",\"type\":\"foundation.mechanical.translational.translational\"}],\"Top\":[]}"
  Translational Damper : fl_lib/Mechanical/Translational Elements/Translational Damper  D=2000 N*s/m  v_specify=off  v_priority=None  v=0 m/s  v_nominal_specify=off  v_nominal_value=1  v_nominal_unit=m/s  f_specify=off  f_priority=None  f=0 N  f_nominal_specify=off  f_nominal_value=1  f_nominal_unit=N
  Translational Spring1 : fl_lib/Mechanical/Translational Elements/Translational Spring  spr_rate=20000 N/m  v_specify=off  v_priority=None  v=0 m/s  v_nominal_specify=off  v_nominal_value=1  v_nominal_unit=m/s  f_specify=off  f_priority=None  f=0 N  f_nominal_specify=off  f_nominal_value=1  f_nominal_unit=N  x_specify=off  x_priority=High  x=0 m  x_nominal_specify=off  x_nominal_value=1  x_nominal_unit=m
  Conn1 : PMIOPort  Side=Right
  Conn2 : PMIOPort  Port=2  Side=Left
  connections:
  Conn2/RConn1 -- Translational Damper/LConn1 -- Translational Inerter/LConn1 -- Translational Spring1/LConn1
  Translational Inerter/RConn1 -- Conn1/RConn1 -- Translational Damper/RConn1 -- Translational Spring1/RConn1

== system RL_sus_quarter_sim/Quarter_sys/Control/Y_1/P_1/Subsystem/p1_k5 ==
  Translational Inerter : fl_lib/Mechanical/Translational Elements/Translational Inerter  B=1 kg  v_specify=off  v_priority=High  v=0 m/s  v_nominal_specify=off  v_nominal_value=1  v_nominal_unit=m/s  f_specify=off  f_priority=None  f=0 N  f_nominal_specify=off  f_nominal_value=1  f_nominal_unit=N
      settings: InternalSimscapePortConfiguration="{\"Bottom\":[],\"Left\":[{\"id\":\"R\",\"label\":\"R\",\"type\":\"foundation.mechanical.translational.translational\"}],\"Right\":[{\"id\":\"C\",\"label\":\"C\",\"type\":\"foundation.mechanical.translational.translational\"}],\"Top\":[]}"
  Translational Damper : fl_lib/Mechanical/Translational Elements/Translational Damper  D=2000 N*s/m  v_specify=off  v_priority=None  v=0 m/s  v_nominal_specify=off  v_nominal_value=1  v_nominal_unit=m/s  f_specify=off  f_priority=None  f=0 N  f_nominal_specify=off  f_nominal_value=1  f_nominal_unit=N
  Translational Spring1 : fl_lib/Mechanical/Translational Elements/Translational Spring  spr_rate=20000 N/m  v_specify=off  v_priority=None  v=0 m/s  v_nominal_specify=off  v_nominal_value=1  v_nominal_unit=m/s  f_specify=off  f_priority=None  f=0 N  f_nominal_specify=off  f_nominal_value=1  f_nominal_unit=N  x_specify=off  x_priority=High  x=0 m  x_nominal_specify=off  x_nominal_value=1  x_nominal_unit=m
  Conn1 : PMIOPort  Side=Right
  Conn2 : PMIOPort  Port=2  Side=Left
  connections:
  Translational Spring1/RConn1 -- Conn1/RConn1
  Translational Inerter/RConn1 -- Translational Spring1/LConn1 -- Translational Damper/RConn1
  Translational Inerter/LConn1 -- Conn2/RConn1 -- Translational Damper/LConn1

== system RL_sus_quarter_sim/Quarter_sys/Control/Y_1/P_1/Subsystem/passive ==
  Translational Damper : fl_lib/Mechanical/Translational Elements/Translational Damper  D=2000 N*s/m  v_specify=off  v_priority=None  v=0 m/s  v_nominal_specify=off  v_nominal_value=1  v_nominal_unit=m/s  f_specify=off  f_priority=None  f=0 N  f_nominal_specify=off  f_nominal_value=1  f_nominal_unit=N
  Translational Spring1 : fl_lib/Mechanical/Translational Elements/Translational Spring  spr_rate=200000 N/m  v_specify=off  v_priority=None  v=0 m/s  v_nominal_specify=off  v_nominal_value=1  v_nominal_unit=m/s  f_specify=off  f_priority=None  f=0 N  f_nominal_specify=off  f_nominal_value=1  f_nominal_unit=N  x_specify=off  x_priority=High  x=0 m  x_nominal_specify=off  x_nominal_value=1  x_nominal_unit=m
  Conn1 : PMIOPort  Side=Right
  Conn2 : PMIOPort  Port=2  Side=Left
  connections:
  Translational Spring1/LConn1 -- Translational Damper/LConn1 -- Conn2/RConn1
  Conn1/RConn1 -- Translational Spring1/RConn1 -- Translational Damper/RConn1

== system RL_sus_quarter_sim/Quarter_sys/Control/Y_1/P_test/Subsystem/p1_k1 ==
  Translational Inerter : fl_lib/Mechanical/Translational Elements/Translational Inerter  B=1 kg  v_specify=off  v_priority=High  v=0 m/s  v_nominal_specify=off  v_nominal_value=1  v_nominal_unit=m/s  f_specify=off  f_priority=None  f=0 N  f_nominal_specify=off  f_nominal_value=1  f_nominal_unit=N
      settings: InternalSimscapePortConfiguration="{\"Bottom\":[],\"Left\":[{\"id\":\"R\",\"label\":\"R\",\"type\":\"foundation.mechanical.translational.translational\"}],\"Right\":[{\"id\":\"C\",\"label\":\"C\",\"type\":\"foundation.mechanical.translational.translational\"}],\"Top\":[]}"
  Translational Damper : fl_lib/Mechanical/Translational Elements/Translational Damper  D=2000 N*s/m  v_specify=off  v_priority=None  v=0 m/s  v_nominal_specify=off  v_nominal_value=1  v_nominal_unit=m/s  f_specify=off  f_priority=None  f=0 N  f_nominal_specify=off  f_nominal_value=1  f_nominal_unit=N
  Translational Spring1 : fl_lib/Mechanical/Translational Elements/Translational Spring  spr_rate=20000 N/m  v_specify=off  v_priority=None  v=0 m/s  v_nominal_specify=off  v_nominal_value=1  v_nominal_unit=m/s  f_specify=off  f_priority=None  f=0 N  f_nominal_specify=off  f_nominal_value=1  f_nominal_unit=N  x_specify=off  x_priority=High  x=0 m  x_nominal_specify=off  x_nominal_value=1  x_nominal_unit=m
  Conn1 : PMIOPort  Side=Right
  Conn2 : PMIOPort  Port=2  Side=Left
  connections:
  Translational Inerter/LConn1 -- Translational Damper/LConn1 -- Conn2/RConn1
  Translational Spring1/LConn1 -- Translational Inerter/RConn1
  Translational Spring1/RConn1 -- Translational Damper/RConn1 -- Conn1/RConn1

== system RL_sus_quarter_sim/Quarter_sys/Control/Y_1/P_test/Subsystem/p1_k2 ==
  Translational Inerter : fl_lib/Mechanical/Translational Elements/Translational Inerter  B=1 kg  v_specify=off  v_priority=High  v=0 m/s  v_nominal_specify=off  v_nominal_value=1  v_nominal_unit=m/s  f_specify=off  f_priority=None  f=0 N  f_nominal_specify=off  f_nominal_value=1  f_nominal_unit=N
      settings: InternalSimscapePortConfiguration="{\"Bottom\":[],\"Left\":[{\"id\":\"R\",\"label\":\"R\",\"type\":\"foundation.mechanical.translational.translational\"}],\"Right\":[{\"id\":\"C\",\"label\":\"C\",\"type\":\"foundation.mechanical.translational.translational\"}],\"Top\":[]}"
  Translational Damper : fl_lib/Mechanical/Translational Elements/Translational Damper  D=2000 N*s/m  v_specify=off  v_priority=None  v=0 m/s  v_nominal_specify=off  v_nominal_value=1  v_nominal_unit=m/s  f_specify=off  f_priority=None  f=0 N  f_nominal_specify=off  f_nominal_value=1  f_nominal_unit=N
  Translational Spring1 : fl_lib/Mechanical/Translational Elements/Translational Spring  spr_rate=20000 N/m  v_specify=off  v_priority=None  v=0 m/s  v_nominal_specify=off  v_nominal_value=1  v_nominal_unit=m/s  f_specify=off  f_priority=None  f=0 N  f_nominal_specify=off  f_nominal_value=1  f_nominal_unit=N  x_specify=off  x_priority=High  x=0 m  x_nominal_specify=off  x_nominal_value=1  x_nominal_unit=m
  Conn1 : PMIOPort  Side=Right
  Conn2 : PMIOPort  Port=2  Side=Left
  connections:
  Translational Damper/RConn1 -- Translational Spring1/LConn1 -- Translational Inerter/RConn1
  Translational Spring1/RConn1 -- Conn1/RConn1
  Conn2/RConn1 -- Translational Damper/LConn1 -- Translational Inerter/LConn1

== system RL_sus_quarter_sim/Quarter_sys/Control/Y_1/P_test/Subsystem/p1_k3 ==
  Translational Inerter : fl_lib/Mechanical/Translational Elements/Translational Inerter  B=1 kg  v_specify=off  v_priority=High  v=0 m/s  v_nominal_specify=off  v_nominal_value=1  v_nominal_unit=m/s  f_specify=off  f_priority=None  f=0 N  f_nominal_specify=off  f_nominal_value=1  f_nominal_unit=N
      settings: InternalSimscapePortConfiguration="{\"Bottom\":[],\"Left\":[{\"id\":\"R\",\"label\":\"R\",\"type\":\"foundation.mechanical.translational.translational\"}],\"Right\":[{\"id\":\"C\",\"label\":\"C\",\"type\":\"foundation.mechanical.translational.translational\"}],\"Top\":[]}"
  Translational Damper : fl_lib/Mechanical/Translational Elements/Translational Damper  D=2000 N*s/m  v_specify=off  v_priority=None  v=0 m/s  v_nominal_specify=off  v_nominal_value=1  v_nominal_unit=m/s  f_specify=off  f_priority=None  f=0 N  f_nominal_specify=off  f_nominal_value=1  f_nominal_unit=N
  Translational Spring1 : fl_lib/Mechanical/Translational Elements/Translational Spring  spr_rate=20000 N/m  v_specify=off  v_priority=None  v=0 m/s  v_nominal_specify=off  v_nominal_value=1  v_nominal_unit=m/s  f_specify=off  f_priority=None  f=0 N  f_nominal_specify=off  f_nominal_value=1  f_nominal_unit=N  x_specify=off  x_priority=High  x=0 m  x_nominal_specify=off  x_nominal_value=1  x_nominal_unit=m
  Conn1 : PMIOPort  Side=Right
  Conn2 : PMIOPort  Port=2  Side=Left
  connections:
  Translational Spring1/RConn1 -- Translational Damper/RConn1 -- Conn1/RConn1 -- Translational Inerter/RConn1
  Translational Spring1/LConn1 -- Translational Inerter/LConn1 -- Translational Damper/LConn1 -- Conn2/RConn1

== system RL_sus_quarter_sim/Quarter_sys/Control/Y_1/P_test/Subsystem/p1_k5 ==
  Translational Inerter : fl_lib/Mechanical/Translational Elements/Translational Inerter  B=1 kg  v_specify=off  v_priority=High  v=0 m/s  v_nominal_specify=off  v_nominal_value=1  v_nominal_unit=m/s  f_specify=off  f_priority=None  f=0 N  f_nominal_specify=off  f_nominal_value=1  f_nominal_unit=N
      settings: InternalSimscapePortConfiguration="{\"Bottom\":[],\"Left\":[{\"id\":\"R\",\"label\":\"R\",\"type\":\"foundation.mechanical.translational.translational\"}],\"Right\":[{\"id\":\"C\",\"label\":\"C\",\"type\":\"foundation.mechanical.translational.translational\"}],\"Top\":[]}"
  Translational Damper : fl_lib/Mechanical/Translational Elements/Translational Damper  D=2000 N*s/m  v_specify=off  v_priority=None  v=0 m/s  v_nominal_specify=off  v_nominal_value=1  v_nominal_unit=m/s  f_specify=off  f_priority=None  f=0 N  f_nominal_specify=off  f_nominal_value=1  f_nominal_unit=N
  Translational Spring1 : fl_lib/Mechanical/Translational Elements/Translational Spring  spr_rate=20000 N/m  v_specify=off  v_priority=None  v=0 m/s  v_nominal_specify=off  v_nominal_value=1  v_nominal_unit=m/s  f_specify=off  f_priority=None  f=0 N  f_nominal_specify=off  f_nominal_value=1  f_nominal_unit=N  x_specify=off  x_priority=High  x=0 m  x_nominal_specify=off  x_nominal_value=1  x_nominal_unit=m
  Conn1 : PMIOPort  Side=Right
  Conn2 : PMIOPort  Port=2  Side=Left
  connections:
  Translational Damper/LConn1 -- Conn2/RConn1 -- Translational Inerter/LConn1
  Translational Damper/RConn1 -- Translational Spring1/LConn1 -- Translational Inerter/RConn1
  Translational Spring1/RConn1 -- Conn1/RConn1

== system RL_sus_quarter_sim/Quarter_sys/Control/Y_1/P_test/Subsystem/passive ==
  Translational Damper : fl_lib/Mechanical/Translational Elements/Translational Damper  D=2000 N*s/m  v_specify=off  v_priority=None  v=0 m/s  v_nominal_specify=off  v_nominal_value=1  v_nominal_unit=m/s  f_specify=off  f_priority=None  f=0 N  f_nominal_specify=off  f_nominal_value=1  f_nominal_unit=N
  Translational Spring1 : fl_lib/Mechanical/Translational Elements/Translational Spring  spr_rate=200000 N/m  v_specify=off  v_priority=None  v=0 m/s  v_nominal_specify=off  v_nominal_value=1  v_nominal_unit=m/s  f_specify=off  f_priority=None  f=0 N  f_nominal_specify=off  f_nominal_value=1  f_nominal_unit=N  x_specify=off  x_priority=High  x=0 m  x_nominal_specify=off  x_nominal_value=1  x_nominal_unit=m
  Conn1 : PMIOPort  Side=Right
  Conn2 : PMIOPort  Port=2  Side=Left
  connections:
  Translational Damper/RConn1 -- Translational Spring1/RConn1 -- Conn1/RConn1
  Conn2/RConn1 -- Translational Damper/LConn1 -- Translational Spring1/LConn1

== system RL_sus_quarter_sim/Quarter_sys/Control/Y_1/Pabbkk/Subsystem/p1_k1 ==
  Translational Inerter : fl_lib/Mechanical/Translational Elements/Translational Inerter  B=1 kg  v_specify=off  v_priority=High  v=0 m/s  v_nominal_specify=off  v_nominal_value=1  v_nominal_unit=m/s  f_specify=off  f_priority=None  f=0 N  f_nominal_specify=off  f_nominal_value=1  f_nominal_unit=N
      settings: InternalSimscapePortConfiguration="{\"Bottom\":[],\"Left\":[{\"id\":\"R\",\"label\":\"R\",\"type\":\"foundation.mechanical.translational.translational\"}],\"Right\":[{\"id\":\"C\",\"label\":\"C\",\"type\":\"foundation.mechanical.translational.translational\"}],\"Top\":[]}"
  Translational Damper : fl_lib/Mechanical/Translational Elements/Translational Damper  D=2000 N*s/m  v_specify=off  v_priority=None  v=0 m/s  v_nominal_specify=off  v_nominal_value=1  v_nominal_unit=m/s  f_specify=off  f_priority=None  f=0 N  f_nominal_specify=off  f_nominal_value=1  f_nominal_unit=N
  Translational Spring1 : fl_lib/Mechanical/Translational Elements/Translational Spring  spr_rate=20000 N/m  v_specify=off  v_priority=None  v=0 m/s  v_nominal_specify=off  v_nominal_value=1  v_nominal_unit=m/s  f_specify=off  f_priority=None  f=0 N  f_nominal_specify=off  f_nominal_value=1  f_nominal_unit=N  x_specify=off  x_priority=High  x=0 m  x_nominal_specify=off  x_nominal_value=1  x_nominal_unit=m
  Conn1 : PMIOPort  Side=Right
  Conn2 : PMIOPort  Port=2  Side=Left
  connections:
  Translational Inerter/LConn1 -- Translational Damper/LConn1 -- Conn2/RConn1
  Translational Spring1/LConn1 -- Translational Inerter/RConn1
  Translational Spring1/RConn1 -- Translational Damper/RConn1 -- Conn1/RConn1
